simulink model "control_simu_disturbance"  (R2024a)
settings: Solver=ode45  StartTime=0.0  StopTime=30  MaxStep=0.001  MinStep=0.00000001
undefined symbols (not defined in the file): K1, Kd, Ke, Ki, Kp, pulse
libraries: fuzblock x1, slpidlib x1, SignalEditorBlockLib x1, simulink x1
settings Model: VariantFading=off  Creator=mainuser  LastModifiedBy=mainuser

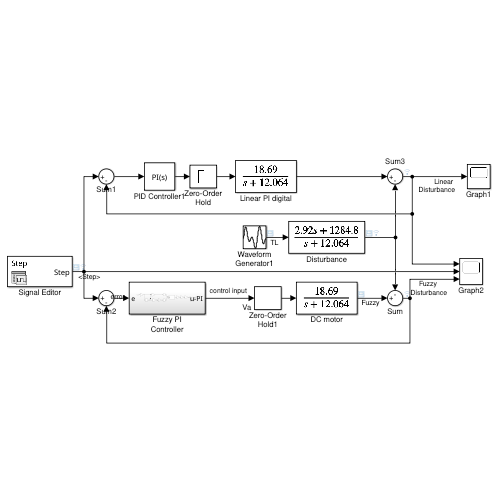
[thumbnail: Simulink's stored preview of the top-level diagram]
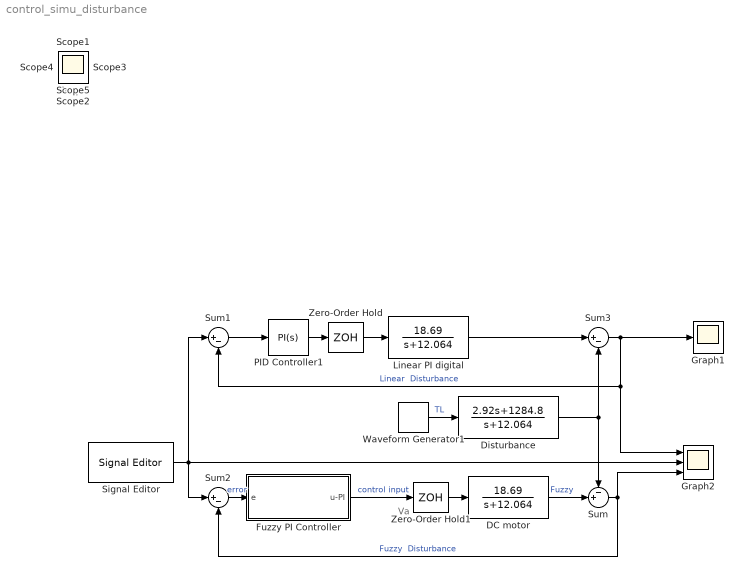
== system control_simu_disturbance ==
  note: Va
  DC motor : TransferFcn  Numerator=[18.69]  Denominator=[1 12.064]
  Disturbance : TransferFcn  Numerator=[2.92 1284.8]  Denominator=[1 12.064]
  Fuzzy PI Controller : Subsystem
  Graph1 : Scope
  Graph2 : Scope  NumInputPorts=3
  Linear PI digital : TransferFcn  Numerator=[18.69]  Denominator=[1 12.064]
  PID Controller1 : slpidlib/PID Controller  Controller=PI  Form=Parallel  TimeDomain=Continuous-time  UseExternalTs=off  SampleTime=-1  IntegratorMethod=Forward Euler  FilterMethod=Forward Euler  ControllerParametersSource=internal  P=Kp  I=Ki  UseKiTs=off  D=0  UseExternalDerivativeSource=off  N=100  UseFilter=on  TunerSelectOption=Transfer Function Based (PID Tuner App)  InitialConditionSource=internal  InitialConditionForIntegrator=0  InitialConditionForFilter=0  DifferentiatorICPrevScaledInput=0  ExternalReset=none  TrackingMode=off  Kt=1  LimitOutput=off  SatLimitsSource=internal  UpperSaturationLimit=inf  LowerSaturationLimit=-inf  LinearizeAsGain=on  AntiWindupMode=none  Kb=1  LimitIntegrator=off  UpperIntegratorSaturationLimit=inf  LowerIntegratorSaturationLimit=-inf  POutMin=[]  POutMax=[]  IOutMin=[]  IOutMax=[]  DOutMin=[]  DOutMax=[]  NOutMin=[]  NOutMax=[]  SumOutMin=[]  SumOutMax=[]  SaturationOutMin=[]  SaturationOutMax=[]  PParamMin=[]  PParamMax=[]  IParamMin=[]  IParamMax=[]  DParamMin=[]  DParamMax=[]  NParamMin=[]  NParamMax=[]  KbParamMin=[]  KbParamMax=[]  KtParamMin=[]  KtParamMax=[]  KbOutMin=[]  KbOutMax=[]  KtOutMin=[]  KtOutMax=[]  IntegratorOutMin=[]  IntegratorOutMax=[]  FilterOutMin=[]  FilterOutMax=[]  SumI1OutMin=[]  SumI1OutMax=[]  SumI2OutMin=[]  SumI2OutMax=[]  SumI3OutMin=[]  SumI3OutMax=[]  SumI4OutMin=[]  SumI4OutMax=[]  SumDOutMin=[]  SumDOutMax=[]  DifferentiatorOutMin=[]  DifferentiatorOutMax=[]  FilterDiffOutCoefMin=[]  FilterDiffOutCoefMax=[]  ReciprocalOutMin=[]  ReciprocalOutMax=[]  SumDenOutMin=[]  SumDenOutMax=[]  SumNumOutMin=[]  SumNumOutMax=[]  DivideOutMin=[]  DivideOutMax=[]  UdiffTsProdOutMin=[]  UdiffTsProdOutMax=[]  NTsProdOutMin=[]  NTsProdOutMax=[]  UintegralTsProdOutMin=[]  UintegralTsProdOutMax=[]  UngainTsProdOutMin=[]  UngainTsProdOutMax=[]  ClampingZeroOutDataTypeStr=Inherit: Inherit via back propagation  ClampingZeroOutMin=[]  ClampingZeroOutMax=[]  FilterDenConstantOutDataTypeStr=Inherit: Inherit via back propagation  FilterDenConstantOutMin=[]  FilterDenConstantOutMax=[]  PCopyOutDataTypeStr=Inherit: Inherit via back propagation  PCopyOutMin=[]  PCopyOutMax=[]  NCopyOutDataTypeStr=Inherit: Inherit via back propagation  NCopyOutMin=[]  NCopyOutMax=[]  IntegratorContinuousStateAttributes=''  IntegratorStateMustResolveToSignalObject=off  IntegratorRTWStateStorageClass=Auto  FilterContinuousStateAttributes=''  FilterStateMustResolveToSignalObject=off  FilterRTWStateStorageClass=Auto  ParallelPVariant=InternalParameters  IdealPVariant=Disabled  IVariant=InternalParameters  DVariant=Disabled  IntegratorVariant=Continuous  SatVariant=Disabled  AWVariant=Passthrough  PCopyVariant=Disabled  TRVariant=Disabled  FdbkBlocksVariant=Forward  IdealPFdbkVariant=Disabled  SatFdbkVariant=Disabled  DerivativeFilterVariant=Disabled  NVariant=Disabled  NCopyVariant=Disabled_SignalSpec  FilterICVariant=Disabled  IntegratorICVariant=InternalICs  ExternalResetVariant=Disabled  TRSumVariant=Passthrough  SumFdbkVariant=Disabled  SumVariant=Sum_PI  TsampFilterVariant=InternalTs  TsampNgainVariant=Passthrough  TsampIntegralVariant=Disabled_SignalSpec  ExternalSaturationOutDataTypeStr=Inherit: Same as second input  DerivativeSourceVariant=Disabled
  Signal Editor : SignalEditorBlockLib/Signal Editor  FileName=scenarios.mat  ActiveScenario=Step  ActiveSignal=Step  IsBus=off  OutputBusObjectStr=Bus: BusObject  SampleTime=0  OutputAfterFinalValue=Holding final value  Unit=inherit  PreserveSignalName=on  ApplySigPropsToAllScenarios=on  ApplySigPropsToAllSignals=off
  Sum : Sum  Inputs=-+|
  Sum1 : Sum  Inputs=|+-
  Sum2 : Sum  Inputs=|+-
  Sum3 : Sum  Inputs=|+-
  Waveform Generator1 : simulink/Sources/Waveform Generator  OutMin=[]  OutMax=[]  OutDataTypeStr=double  SelectedSignal=1  Signals=0.5+pulse('Amplitude',0.5,'TriggerTime',10,'Duration',9.95)  BlockNames=MultiportSwitch_e785c34bd2c5499  SampleTime=0.1
  Zero-Order Hold : ZeroOrderHold  SampleTime=0.01
  Zero-Order Hold1 : ZeroOrderHold  SampleTime=0.01
  Scope{,1..5} (6 alike) : Scope
  wires:
  Sum1/1 -> PID Controller1/1
  Linear PI digital/1 -> Sum3/1
  PID Controller1/1 -> Zero-Order Hold/1
  Zero-Order Hold/1 -> Linear PI digital/1
  Zero-Order Hold1/1 -> DC motor/1
  Fuzzy PI Controller/1(u-PI) -> Zero-Order Hold1/1  "control input"
  Sum2/1 -> Fuzzy PI Controller/1(e)  "error"
  Signal Editor/1 -> Sum2/1, Graph2/2, Sum1/1
  DC motor/1 -> Sum/2  "Fuzzy"
  Waveform Generator1/1 -> Disturbance/1  "TL"
  Disturbance/1 -> Sum/1, Sum3/2
  Sum/1 -> Sum2/2, Graph2/3  "Fuzzy  Disturbance"
  Sum3/1 -> Graph1/1, Graph2/1, Sum1/2  "Linear  Disturbance"

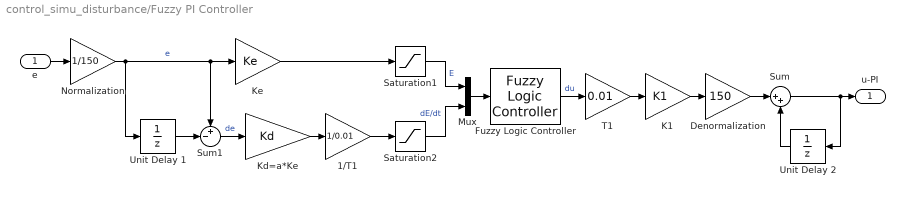
== system control_simu_disturbance/Fuzzy PI Controller ==
  e : Inport
  1/T1 : Gain  Gain=1/0.01
  Denormalization : Gain  Gain=150
  Fuzzy Logic Controller : fuzblock/Fuzzy Logic  Controller  FIS='flb.fis'  OutputSampleNumber=101  DataType=double  FuzzifiedInputs=off  RuleFiringStrengths=off  RuleOutputs=off  AggregatedOutputs=off  SimulateUsing=Interpreted execution  OutOfRangeInputValueMessage=none  NoRuleFiredMessage=warning  EmptyOutputFuzzySetMessage=warning
  K1 : Gain  Gain=K1
  Kd=a*Ke : Gain  Gain=Kd
  Ke : Gain  Gain=Ke
  Mux : Mux  Inputs=2
  Normalization : Gain  Gain=1/150
  Saturation1 : Saturate  UpperLimit=1  LowerLimit=-1
  Saturation2 : Saturate  UpperLimit=1  LowerLimit=-0.97
  Sum : Sum  Inputs=|++
  Sum1 : Sum  Inputs=+-|
  T1 : Gain  Gain=0.01
  Unit Delay 1 : UnitDelay  SampleTime=-1  HasFrameUpgradeWarning=on
  Unit Delay 2 : UnitDelay  SampleTime=-1  HasFrameUpgradeWarning=on
  u-PI : Outport
  wires:
  e/1 -> Normalization/1
  Normalization/1 -> Sum1/1, Ke/1, Unit Delay 1/1  "e"
  Unit Delay 1/1 -> Sum1/2
  Sum1/1 -> Kd=a*Ke/1  "de"
  Kd=a*Ke/1 -> 1/T1/1
  Ke/1 -> Saturation1/1
  1/T1/1 -> Saturation2/1
  Saturation1/1 -> Mux/1  "E"
  Saturation2/1 -> Mux/2  "dE/dt"
  Mux/1 -> Fuzzy Logic Controller/1
  Fuzzy Logic Controller/1 -> T1/1  "du"
  T1/1 -> K1/1
  K1/1 -> Denormalization/1
  Denormalization/1 -> Sum/1
  Unit Delay 2/1 -> Sum/2
  Sum/1 -> Unit Delay 2/1, u-PI/1
